simulink model "simulation1"  (R2021b)
settings: Solver=VariableStepAuto  StartTime=0.0  StopTime=10.0  RelTol=1e-3
values from neighbouring files (symbols this model uses):
  B = 0.03    [dcmotor_parameters.m]    (also in simulation.m = 0.01)
  KePhi = 1.6    [dcmotor_parameters.m]    (also in simulation.m)
  Ra = 1    [dcmotor_parameters.m]    (also in simulation.m = 0.5)
  tau_a = La/Ra    (= 0.2)    [dcmotor_parameters.m]    (also in simulation.m)
  tau_m = J/B    (= 266.666666667)    [dcmotor_parameters.m]    (also in simulation.m = 500)
  TL = 0    [dcmotor_parameters.m]    (also in simulation.m = 20)
  Va = 12    [dcmotor_parameters.m]    (also in simulation.m)
libraries: simulink_extras x2
settings Model: Creator=sacka  LastModifiedBy=sacka

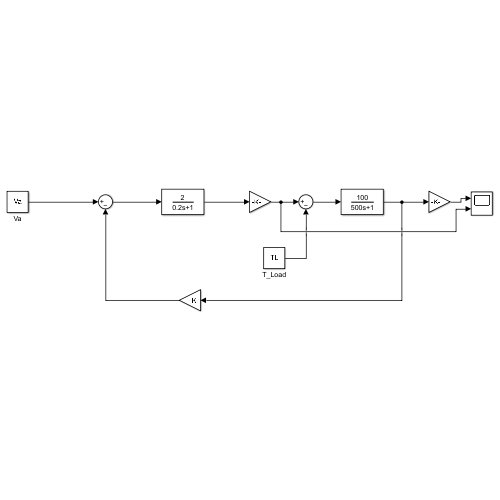
[thumbnail: Simulink's stored preview of the top-level diagram]
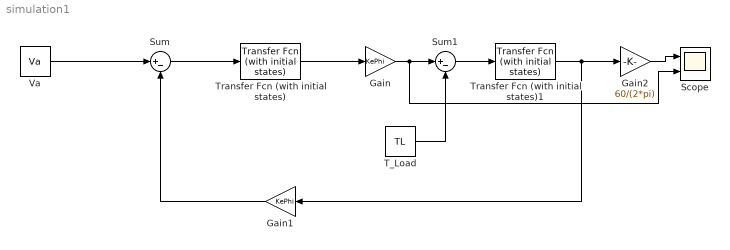
== system simulation1 ==
  Gain : Gain  Gain=KePhi
  Gain1 : Gain  Gain=KePhi
  Gain2 : Gain  Gain=60/(2*pi)
  Scope : Scope  NumInputPorts=2
  Sum : Sum  Inputs=|+-
  Sum1 : Sum  Inputs=|+-
  T_Load : Constant  Value=TL
  Transfer Fcn (with initial states) : simulink_extras/Additional Linear/Transfer Fcn (with initial states)  N=[1/Ra]  D=[tau_a 1]  X0=.5
  Transfer Fcn (with initial states)1 : simulink_extras/Additional Linear/Transfer Fcn (with initial states)  N=[1/B]  D="[tau_m  1]"  X0=.5
  Va : Constant  Value=Va
  wires:
  Va/1 -> Sum/1
  Sum/1 -> Transfer Fcn (with initial states)/1
  Transfer Fcn (with initial states)/1 -> Gain/1
  Gain/1 -> Scope/2, Sum1/1
  T_Load/1 -> Sum1/2
  Sum1/1 -> Transfer Fcn (with initial states)1/1
  Transfer Fcn (with initial states)1/1 -> Gain2/1, Gain1/1
  Gain1/1 -> Sum/2
  Gain2/1 -> Scope/1
